simulink model "drone"  (R2022a)
settings: Solver=FixedStepAuto  StartTime=0.0  StopTime=20  FixedStep=1  RelTol=1e-3
settings Model: Creator=JadKHaddad  LastModifiedBy=JadKHaddad

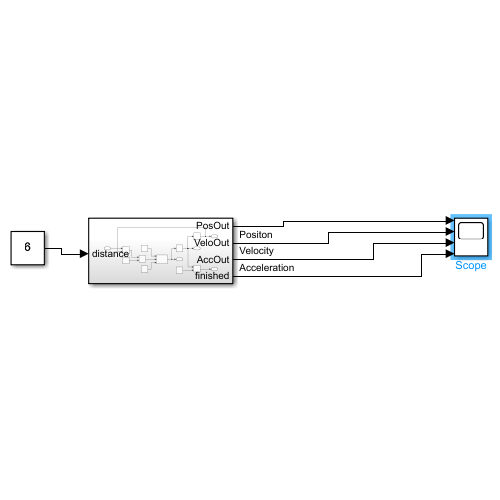
[thumbnail: Simulink's stored preview of the top-level diagram]
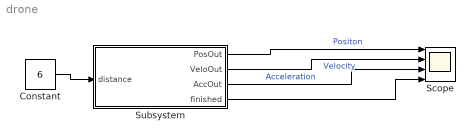
== system drone ==
  Constant : Constant  Value=6
  Scope : Scope  NumInputPorts=4
  Subsystem : Subsystem
  wires:
  Subsystem/2(VeloOut) -> Scope/2  "Velocity"
  Subsystem/3(AccOut) -> Scope/3  "Acceleration"
  Constant/1 -> Subsystem/1(distance)
  Subsystem/1(PosOut) -> Scope/1  "Positon"
  Subsystem/4(finished) -> Scope/4

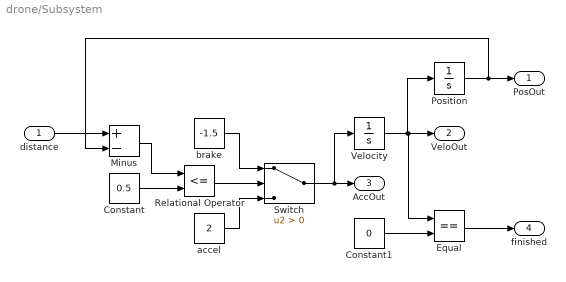
== system drone/Subsystem ==
  distance : Inport
  Constant : Constant  Value=0.5
  Constant1 : Constant  Value=0
  Equal : RelationalOperator  Operator===  OutDataTypeStr=boolean  RndMeth=Simplest  InputSameDT=off
  Minus : Sum  Inputs=+-
  Position : Integrator
  Relational Operator : RelationalOperator  Operator=<=  OutDataTypeStr=boolean  RndMeth=Simplest  InputSameDT=off
  Switch : Switch  Criteria=u2 > Threshold  SaturateOnIntegerOverflow=off  InputSameDT=off
  Velocity : Integrator  LimitOutput=on  UpperSaturationLimit=1  LowerSaturationLimit=0
  accel : Constant  Value=2
  brake : Constant  Value=-1.5
  PosOut : Outport
  VeloOut : Outport  Port=2
  AccOut : Outport  Port=3
  finished : Outport  Port=4
  wires:
  Constant/1 -> Relational Operator/2
  distance/1 -> Minus/1
  Constant1/1 -> Equal/2
  Relational Operator/1 -> Switch/2
  Equal/1 -> finished/1
  Minus/1 -> Relational Operator/1
  Switch/1 -> Velocity/1, AccOut/1
  brake/1 -> Switch/1
  accel/1 -> Switch/3
  Velocity/1 -> VeloOut/1, Equal/1, Position/1
  Position/1 -> Minus/2, PosOut/1
